simulink model "DC_6a_es"  (R2022b)
settings: Solver=VariableStepAuto  StartTime=0.0  StopTime=10.0  RelTol=1e-3
undefined symbols (not defined in the file or in its folder): ts
libraries: cstblocks x2
settings Model: Creator=alici  LastModifiedBy=alici

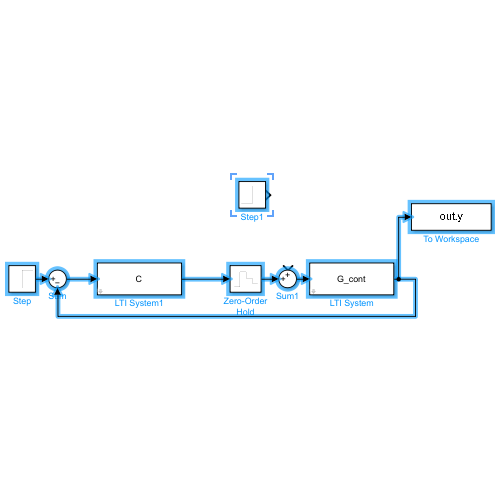
[thumbnail: Simulink's stored preview of the top-level diagram]
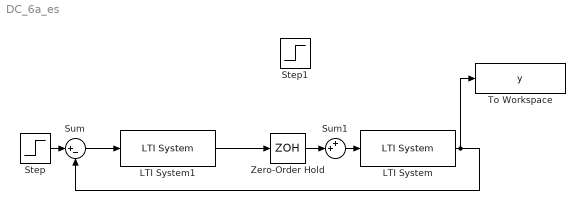
== system DC_6a_es ==
  LTI System : cstblocks/LTI System  sys=G_cont  IC=[]
  LTI System1 : cstblocks/LTI System  sys=C  IC=[]
  Step : Step  Time=0  SampleTime=0
  Step1 : Step  Time=0  SampleTime=0
  Sum : Sum  Inputs=|+-
  Sum1 : Sum  Inputs=++|
  To Workspace : ToWorkspace  VariableName=y  SaveFormat=Timeseries  SampleTime=ts/1000
  Zero-Order Hold : ZeroOrderHold  SampleTime=ts
  wires:
  LTI System1/1 -> Zero-Order Hold/1
  Zero-Order Hold/1 -> Sum1/2
  Sum1/1 -> LTI System/1
  Sum/1 -> LTI System1/1
  LTI System/1 -> To Workspace/1, Sum/2
  Step/1 -> Sum/1
